simulink subsystem "Controller"  (R2025a)
settings: Solver=VariableStepAuto  StartTime=0.0  StopTime=10.0  RelTol=1e-3
undefined symbols (not defined in the file): Kd, Kp
settings Model: Creator=Jackt  LastModifiedBy=Jackt

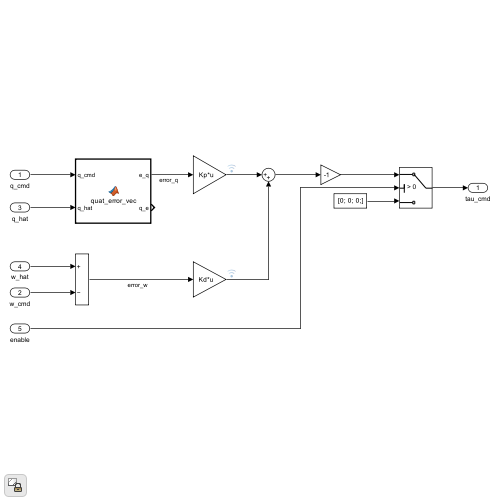
[thumbnail: Simulink's stored preview of the top-level diagram]
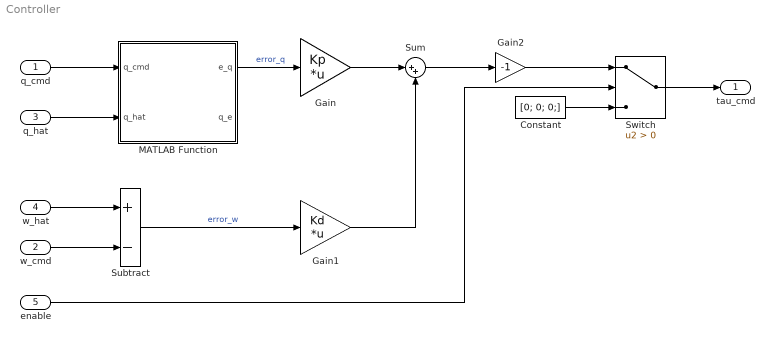
== system Controller ==
  q_cmd : Inport
  w_cmd : Inport  Port=2
  q_hat : Inport  Port=3
  w_hat : Inport  Port=4
  enable : Inport  Port=5
  Constant : Constant  Value=[0; 0; 0;]
  Gain : Gain  Gain=Kp  Multiplication=Matrix(K*u)
  Gain1 : Gain  Gain=Kd  Multiplication=Matrix(K*u)
  Gain2 : Gain  Gain=-1
  MATLAB Function : MATLAB Function  TreatAsAtomicUnit=on
  Subtract : Sum  Inputs=+-
  Sum : Sum  Inputs=|++
  Switch : Switch  Criteria=u2 > Threshold  SaturateOnIntegerOverflow=off  InputSameDT=off
  tau_cmd : Outport
  wires:
  q_cmd/1 -> MATLAB Function/1(q_cmd)
  q_hat/1 -> MATLAB Function/2(q_hat)
  w_hat/1 -> Subtract/1
  w_cmd/1 -> Subtract/2
  MATLAB Function/1(e_q) -> Gain/1  "error_q"
  Subtract/1 -> Gain1/1  "error_w"
  Gain/1 -> Sum/1
  Sum/1 -> Gain2/1
  Gain1/1 -> Sum/2
  enable/1 -> Switch/2
  Constant/1 -> Switch/3
  Switch/1 -> tau_cmd/1
  Gain2/1 -> Switch/1

== matlab function Controller/MATLAB Function ==
  data: q_cmd input; e_q output; q_hat input; q_e output
function [e_q, q_e] = quat_error_vec(q_cmd, q_hat)
%Calculate quaternion inverse (assume scalar first)
q_star = [q_cmd(1); -q_cmd(2); -q_cmd(3); -q_cmd(4)];
q_cmd_inv = q_star / norm(q_star)^2;

%Calculate q_e via hamilton product
q_e = quat_mul(q_cmd_inv, q_hat);

%Force quaternion to take the shortest route
if(q_e(1) < 0)
    q_e = -q_e;
end

%Convert to axis angle with log-mapping
s = q_e(1); %Scalar part
v = q_e(2:4); %Vector part
r = norm(v);

theta = 2 * atan2(r, s);

eps_r = 1e-9; %Machine precision
if(r < eps_r)
    e_q = [0; 0; 0]
else %If near machine precision
    e_q = theta * (v/r);
end

end

function q = quat_mul(p, r)
% p ⊗ r, both scalar-first
p0 = p(1); pv = p(2:4);
r0 = r(1); rv = r(2:4);

q0 = p0*r0 - dot(pv, rv);
qv = p0*rv + r0*pv + cross(pv, rv);

q = [q0; qv];
end
